simulink model "basicKin_sim1"  (R2025a)
settings: Solver=FixedStepDiscrete  StartTime=0.0  StopTime=1  FixedStep=TS  RelTol=1e-3  EnableMultiTasking=on
PostLoadFcn:
  | paramsBasicKinematics
model workspace (MAT data in the model file):
  Ia = 0.1
  Id = 0.25
  Pa = 5
  Pd = 9
  TS = 0.01
settings Model: Creator=mgovinda  LastModifiedBy=garellan
settings SolverCC: AlgebraicLoopSolver=TrustRegion
settings DataIOCC: LimitDataPoints=on  SaveFormat=Array  ReturnWorkspaceOutputs=off
settings OptimizationCC: LifeSpan=inf
settings DebuggingCC: UnconnectedInputMsg=warning  UnconnectedOutputMsg=warning  UnconnectedLineMsg=warning  SFUnexpectedBacktrackingDiag=warning  SFNoUnconditionalDefaultTransitionDiag=warning  SFExecutionAtInitializationDiag=none  ArithmeticOperatorsInVariantConditions=warning
settings HardwareCC: ProdBitPerPointer=32.0  ProdBitPerSizeT=32.0  ProdBitPerPtrDiffT=32.0  ProdLargestAtomicFloat=None  ProdIntDivRoundTo=Undefined  ProdEndianess=Unspecified  ProdWordSize=32.0  ProdHWDeviceType=32-bit Generic
settings ModelReferenceCC: EnableRefExpFcnMdlSchedulingChecks=on  PropagateSignalLabelsOutOfModel=off
settings SFSimCC: SimUseLocalCustomCode=off  CustomCodeUndefinedFunction=UseInterfaceOnly
settings RTWCC: RTWUseLocalCustomCode=off  GPUComputeCapability=3.5  DLArmComputeVersion=19.05
settings CodeAppCC: StateflowObjectComments=on
settings GRTTargetCC: TargetLangStandard=C89/C90 (ANSI)
settings ConfigComp: CovMetricSettings=dw  CovSaveCumulativeToWorkspaceVar=on  CovSaveSingleToWorkspaceVar=on  CovExternalEMLEnable=off

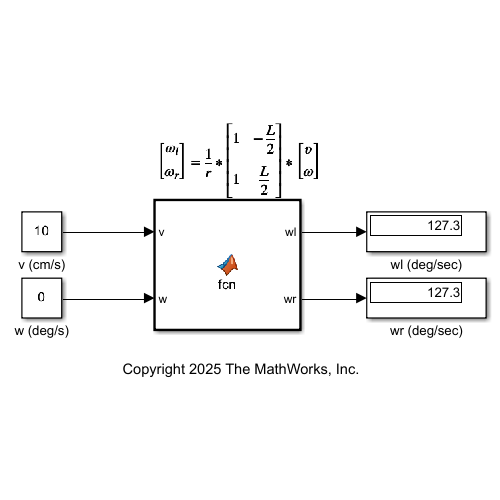
[thumbnail: Simulink's stored preview of the top-level diagram]
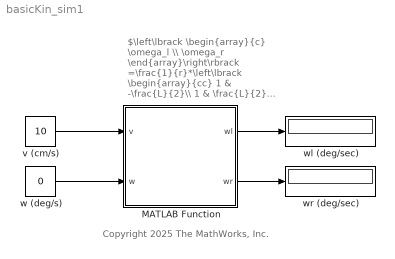
== system basicKin_sim1 ==
  note: Copyright 2025 The MathWorks, Inc.
  note: $\left\lbrack \begin{array}{c} \omega_l \\ \omega_r \end{array}\right\rbrack =\frac{1}{r}*\left\lbrack \begin{array}{cc} 1 & -\frac{L}{2}\\ 1 & \frac{L}{2} \end{array}\right\rbrack *\left\lbrack \begin{array}{c} \upsilon \\ \omega \end{array}\right\rbrack$
  MATLAB Function : MATLAB Function  TreatAsAtomicUnit=on
  "v (cm/s) " : Constant  Value=10
  w (deg/s) : Constant  Value=0
  wl (deg/sec) : Display
  wr (deg/sec) : Display
  wires:
  MATLAB Function/1(wl) -> wl (deg/sec)/1
  MATLAB Function/2(wr) -> wr (deg/sec)/1
  "v (cm/s) "/1 -> MATLAB Function/1(v)
  w (deg/s)/1 -> MATLAB Function/2(w)

== matlab function basicKin_sim1/MATLAB Function ==
  data: v input; wl output; w input; wr output
function [wl,wr] = fcn(v,w)

%FCN Calculates wheel speeds wl and wr
%   v: Rover velocity
%   w: Rate of rotation

L = 8.8; % Length
r = 4.5; % Wheel radius
w = w*pi/180; 

wheelVels = 1/r*[1 -L/2; 1 L/2] * [v;w] *180/pi;
wl = wheelVels(1);
wr = wheelVels(2);
    
end
